simulink library "Contact_Forces_Lib"  (R2018a)
settings: Solver=ode45  StartTime=0.0  StopTime=10.0  RelTol=1e-3  EnableMultiTasking=on
undefined symbols (not defined in the file or in its folder): b_contact, custom_param_1, custom_param_2, k_contact, l_cone, length_cylinder, length_tube, mu_kinetic, mu_static, pen_exponent, pen_full_damp_F, rad_s_cone, radius_cylinder, radius_tube, v_thr, X, Y, Z
libraries: nesl_utility x153, sm_lib x64, $bdroot x53, simulink x9, fl_lib x1
(part 3 of 7)

== system Contact_Forces_Lib/2D/Circle to Circle Force/Fn ==
  note: Resolve Normal Force in
      | Circle F reference frame
  note: Resolve Normal Force in
      | Circle B reference frame
  Fn : Inport
  R : Inport  Port=2
  azm : Inport  Port=3
  Fn in CirB : Subsystem
  Fn in CirF : Subsystem
  FxCirF : Outport
  FyCirF : Outport  Port=2
  FxCirB : Outport  Port=3
  FyCirB : Outport  Port=4
  wires:
  Fn in CirF/2(FxCirF) -> FxCirF/1
  Fn in CirF/1(FyCirF) -> FyCirF/1
  R/1 -> Fn in CirF/1(R)
  azm/1 -> Fn in CirB/2(azm)
  Fn/1 -> Fn in CirB/1(Fn)
  Fn in CirB/2(FyCirB) -> FyCirB/1, Fn in CirF/3(FyCirB)
  Fn in CirB/1(FxCirB) -> Fn in CirF/2(FxCirB), FxCirB/1

== system Contact_Forces_Lib/2D/Circle to Circle Force/Sensing ==
  PS-Simulink Converter1 : nesl_utility/PS-Simulink Converter  PhysicalDomain=network_engine_domain  SubClassName=ps_output  LeftPortType=input  RightPortType=output  PseudoPeriodic=off  Frequencies=[]  Unit=deg  AffineConversion=off
  PS-Simulink Converter{2..7} (6 alike) : nesl_utility/PS-Simulink Converter  PhysicalDomain=network_engine_domain  SubClassName=ps_output  LeftPortType=input  RightPortType=output  PseudoPeriodic=off  Frequencies=[]  Unit=1  AffineConversion=off
  Selector : Selector  NumberOfDimensions=2  InputPortWidth=3  IndexOptions=Index vector (dialog),Index vector (dialog)  Indices=[1,2],[1,2]  OutputSizes=1,1
  Transform Sensor Base : sm_lib/Frames and Transforms/Transform Sensor  MeasurementFrame=Base  SenseAngle=off  SenseAxis=off  SenseAngle1=off  SenseAngle2=off  SenseAngle3=off  SenseQ=off  SenseR=on  SenseOmegaX=off  SenseOmegaY=off  SenseOmegaZ=off  SenseOmega1=off  SenseOmega2=off  SenseOmega3=off  SenseQDot=off  SenseRDot=off  SenseAlphaX=off  SenseAlphaY=off  SenseAlphaZ=off  SenseAlpha1=off  SenseAlpha2=off  SenseAlpha3=off  SenseQDDot=off  SenseRDDot=off  SenseX=off  SenseY=off  SenseZ=off  SenseRad=on  SenseAzim=on  SenseDist=off  SenseInc=off  SenseXDot=off  SenseYDot=off  SenseZDot=off  SenseRadDot=on  SenseAzimDot=off  SenseDistDot=off  SenseIncDot=off  SenseXDDot=off  SenseYDDot=off  SenseZDDot=off  SenseRadDDot=off  SenseAzimDDot=off  SenseDistDDot=off  SenseIncDDot=off  BlockFunction=simmechanics.library.frames_transforms.transform_sensor
  Transform Sensor NonRotBase : sm_lib/Frames and Transforms/Transform Sensor  MeasurementFrame=NonRotatingBase  SenseAngle=off  SenseAxis=off  SenseAngle1=off  SenseAngle2=off  SenseAngle3=off  SenseQ=off  SenseR=off  SenseOmegaX=off  SenseOmegaY=off  SenseOmegaZ=off  SenseOmega1=off  SenseOmega2=off  SenseOmega3=off  SenseQDot=off  SenseRDot=off  SenseAlphaX=off  SenseAlphaY=off  SenseAlphaZ=off  SenseAlpha1=off  SenseAlpha2=off  SenseAlpha3=off  SenseQDDot=off  SenseRDDot=off  SenseX=off  SenseY=off  SenseZ=off  SenseRad=off  SenseAzim=off  SenseDist=off  SenseInc=off  SenseXDot=off  SenseYDot=off  SenseZDot=off  SenseRadDot=off  SenseAzimDot=on  SenseDistDot=off  SenseIncDot=off  SenseXDDot=off  SenseYDDot=off  SenseZDDot=off  SenseRadDDot=off  SenseAzimDDot=off  SenseDistDDot=off  SenseIncDDot=off  BlockFunction=simmechanics.library.frames_transforms.transform_sensor
  Transform Sensor WorldB : sm_lib/Frames and Transforms/Transform Sensor  MeasurementFrame=Follower  SenseAngle=off  SenseAxis=off  SenseAngle1=off  SenseAngle2=off  SenseAngle3=off  SenseQ=off  SenseR=off  SenseOmegaX=off  SenseOmegaY=off  SenseOmegaZ=on  SenseOmega1=off  SenseOmega2=off  SenseOmega3=off  SenseQDot=off  SenseRDot=off  SenseAlphaX=off  SenseAlphaY=off  SenseAlphaZ=off  SenseAlpha1=off  SenseAlpha2=off  SenseAlpha3=off  SenseQDDot=off  SenseRDDot=off  SenseX=off  SenseY=off  SenseZ=off  SenseRad=off  SenseAzim=off  SenseDist=off  SenseInc=off  SenseXDot=off  SenseYDot=off  SenseZDot=off  SenseRadDot=off  SenseAzimDot=off  SenseDistDot=off  SenseIncDot=off  SenseXDDot=off  SenseYDDot=off  SenseZDDot=off  SenseRadDDot=off  SenseAzimDDot=off  SenseDistDDot=off  SenseIncDDot=off  BlockFunction=simmechanics.library.frames_transforms.transform_sensor
  Transform Sensor WorldF : sm_lib/Frames and Transforms/Transform Sensor  MeasurementFrame=Follower  SenseAngle=off  SenseAxis=off  SenseAngle1=off  SenseAngle2=off  SenseAngle3=off  SenseQ=off  SenseR=off  SenseOmegaX=off  SenseOmegaY=off  SenseOmegaZ=on  SenseOmega1=off  SenseOmega2=off  SenseOmega3=off  SenseQDot=off  SenseRDot=off  SenseAlphaX=off  SenseAlphaY=off  SenseAlphaZ=off  SenseAlpha1=off  SenseAlpha2=off  SenseAlpha3=off  SenseQDDot=off  SenseRDDot=off  SenseX=off  SenseY=off  SenseZ=off  SenseRad=off  SenseAzim=off  SenseDist=off  SenseInc=off  SenseXDot=off  SenseYDot=off  SenseZDot=off  SenseRadDot=off  SenseAzimDot=off  SenseDistDot=off  SenseIncDot=off  SenseXDDot=off  SenseYDDot=off  SenseZDDot=off  SenseRadDDot=off  SenseAzimDDot=off  SenseDistDDot=off  SenseIncDDot=off  BlockFunction=simmechanics.library.frames_transforms.transform_sensor
  World Frame1 : sm_lib/Frames and Transforms/World Frame  BlockFunction=simmechanics.library.frames_transforms.world_frame
  F : PMIOPort  Side=Left
  B : PMIOPort  Port=2  Side=Left
  rad : Outport
  vrad : Outport  Port=2
  azm : Outport  Port=3
  vazm : Outport  Port=4
  wzf : Outport  Port=5
  wzb : Outport  Port=6
  R : Outport  Port=7
  wires:
  PS-Simulink Converter7/1 -> wzb/1
  PS-Simulink Converter1/1 -> azm/1
  PS-Simulink Converter5/1 -> rad/1
  PS-Simulink Converter4/1 -> vrad/1
  Selector/1 -> R/1
  PS-Simulink Converter6/1 -> Selector/1
  PS-Simulink Converter2/1 -> vazm/1
  PS-Simulink Converter3/1 -> wzf/1
  connections:
  PS-Simulink Converter7/LConn1 -- Transform Sensor WorldB/RConn2
  Transform Sensor WorldF/LConn1 -- Transform Sensor WorldB/LConn1 -- World Frame1/RConn1
  PS-Simulink Converter4/LConn1 -- Transform Sensor Base/RConn5
  PS-Simulink Converter5/LConn1 -- Transform Sensor Base/RConn3
  PS-Simulink Converter1/LConn1 -- Transform Sensor Base/RConn4
  PS-Simulink Converter6/LConn1 -- Transform Sensor Base/RConn2
  Transform Sensor Base/LConn1 -- B/RConn1 -- Transform Sensor NonRotBase/LConn1 -- Transform Sensor WorldB/RConn1
  Transform Sensor WorldF/RConn1 -- F/RConn1 -- Transform Sensor Base/RConn1 -- Transform Sensor NonRotBase/RConn1
  PS-Simulink Converter2/LConn1 -- Transform Sensor NonRotBase/RConn2
  PS-Simulink Converter3/LConn1 -- Transform Sensor WorldF/RConn2

== system Contact_Forces_Lib/2D/Circle to Circle Force/Sum ==
  FnxCirF : Inport
  FnyCirF : Inport  Port=2
  FnxCirB : Inport  Port=3
  FnyCirB : Inport  Port=4
  FfxCirF : Inport  Port=5
  FfyCirF : Inport  Port=6
  FfxCirB : Inport  Port=7
  FfyCirB : Inport  Port=8
  TzCirF : Inport  Port=9
  TzCirB : Inport  Port=10
  Simulink-PS Converter{,3..7} (6 alike) : nesl_utility/Simulink-PS Converter  PhysicalDomain=network_engine_domain  SubClassName=ps_input  LeftPortType=input  RightPortType=output  PseudoPeriodic=off  Frequencies=[]  NoiseDistribution=none  NoiseParameters=[]  Unit=1  AffineConversion=off  InputFiltering=off  SimscapeFilterOrder=1  InputFilterTimeConstant=.001  UdotUserProvided=[]
  Sum{2..5} (4 alike) : Sum
  FxF : PMIOPort  Side=Right
  FyF : PMIOPort  Port=2  Side=Right
  TzF : PMIOPort  Port=3  Side=Right
  FxB : PMIOPort  Port=4  Side=Right
  FyB : PMIOPort  Port=5  Side=Right
  TzB : PMIOPort  Port=6  Side=Right
  wires:
  FfxCirF/1 -> Sum4/2
  FfyCirF/1 -> Sum2/2
  FfyCirB/1 -> Sum5/2
  FfxCirB/1 -> Sum3/2
  TzCirF/1 -> Simulink-PS Converter6/1
  TzCirB/1 -> Simulink-PS Converter7/1
  FnxCirF/1 -> Sum4/1
  FnyCirF/1 -> Sum2/1
  FnxCirB/1 -> Sum3/1
  FnyCirB/1 -> Sum5/1
  Sum4/1 -> Simulink-PS Converter/1
  Sum2/1 -> Simulink-PS Converter3/1
  Sum3/1 -> Simulink-PS Converter4/1
  Sum5/1 -> Simulink-PS Converter5/1
  connections:
  Simulink-PS Converter/RConn1 -- FxF/RConn1
  Simulink-PS Converter3/RConn1 -- FyF/RConn1
  Simulink-PS Converter4/RConn1 -- FxB/RConn1
  Simulink-PS Converter5/RConn1 -- FyB/RConn1
  Simulink-PS Converter6/RConn1 -- TzF/RConn1
  Simulink-PS Converter7/RConn1 -- TzB/RConn1

== system Contact_Forces_Lib/2D/Circle to Circle Force Enabled/Calculate Penetration ==
  rad : Inport
  vrad : Inport  Port=2
  Constant : Constant  Value=cirF_rad+cirB_rad
  Dead Zone : DeadZone  LowerValue=-inf  UpperValue=0  SaturateOnIntegerOverflow=on
  Gain2 : Gain  Gain=-1
  Sum1 : Sum  Inputs=+-
  Pen : Outport
  Pen Vel : Outport  Port=2
  wires:
  vrad/1 -> Gain2/1
  Gain2/1 -> Pen Vel/1
  Dead Zone/1 -> Pen/1
  Sum1/1 -> Dead Zone/1
  Constant/1 -> Sum1/1
  rad/1 -> Sum1/2

== system Contact_Forces_Lib/2D/Circle to Circle Force Enabled/Ff ==
  Fn : Inport
  azm : Inport  Port=2
  Pen : Inport  Port=3
  rad : Inport  Port=4
  vazm : Inport  Port=5
  wzf : Inport  Port=6
  wzb : Inport  Port=7
  R : Inport  Port=8
  Friction Law : $bdroot/Friction Law  OverrideUsingVariant=None
  Resolve Ff : Subsystem
  vTan : Subsystem
  FxCirF : Outport
  FyCirF : Outport  Port=2
  FxCirB : Outport  Port=3
  FyCirB : Outport  Port=4
  TzCirF : Outport  Port=5
  TzCirB : Outport  Port=6
  Ff : Outport  Port=7
  wires:
  Resolve Ff/6(TzCirB) -> TzCirB/1
  Resolve Ff/5(TzCirF) -> TzCirF/1
  Resolve Ff/2(FyCirB) -> FyCirB/1
  Resolve Ff/1(FxCirB) -> FxCirB/1
  Resolve Ff/3(FyCirF) -> FyCirF/1
  Resolve Ff/4(FxCirF) -> FxCirF/1
  Friction Law/1 -> Ff/1, Resolve Ff/2(Ff)
  vTan/1(vTan) -> Friction Law/2
  wzf/1 -> vTan/4(wzf)
  vazm/1 -> vTan/3(vazm)
  rad/1 -> vTan/1(rad)
  Fn/1 -> Friction Law/1
  Pen/1 -> vTan/2(Pen)
  azm/1 -> Resolve Ff/3(azm)
  R/1 -> Resolve Ff/1(R)
  wzb/1 -> vTan/5(wzb)

== system Contact_Forces_Lib/2D/Circle to Circle Force Enabled/Fn ==
  note: Resolve Normal Force in
      | Circle B reference frame
  note: Resolve Normal Force in
      | Circle F reference frame
  Fn : Inport
  R : Inport  Port=2
  azm : Inport  Port=3
  Fn in CirB : Subsystem
  Fn in CirF : Subsystem
  FxCirF : Outport
  FyCirF : Outport  Port=2
  FxCirB : Outport  Port=3
  FyCirB : Outport  Port=4
  wires:
  Fn in CirB/1(FxCirB) -> FxCirB/1, Fn in CirF/2(FxCirB)
  Fn in CirB/2(FyCirB) -> Fn in CirF/3(FyCirB), FyCirB/1
  Fn/1 -> Fn in CirB/1(Fn)
  azm/1 -> Fn in CirB/2(azm)
  R/1 -> Fn in CirF/1(R)
  Fn in CirF/1(FyCirF) -> FyCirF/1
  Fn in CirF/2(FxCirF) -> FxCirF/1

== system Contact_Forces_Lib/2D/Circle to Circle Force Enabled/Sensing ==
  PS-Simulink Converter1 : nesl_utility/PS-Simulink Converter  PhysicalDomain=network_engine_domain  SubClassName=ps_output  LeftPortType=input  RightPortType=output  PseudoPeriodic=off  Frequencies=[]  Unit=deg  AffineConversion=off
  PS-Simulink Converter{2..7} (6 alike) : nesl_utility/PS-Simulink Converter  PhysicalDomain=network_engine_domain  SubClassName=ps_output  LeftPortType=input  RightPortType=output  PseudoPeriodic=off  Frequencies=[]  Unit=1  AffineConversion=off
  Selector : Selector  NumberOfDimensions=2  InputPortWidth=3  IndexOptions=Index vector (dialog),Index vector (dialog)  Indices=[1,2],[1,2]  OutputSizes=1,1
  Transform Sensor Base : sm_lib/Frames and Transforms/Transform Sensor  MeasurementFrame=Base  SenseAngle=off  SenseAxis=off  SenseAngle1=off  SenseAngle2=off  SenseAngle3=off  SenseQ=off  SenseR=on  SenseOmegaX=off  SenseOmegaY=off  SenseOmegaZ=off  SenseOmega1=off  SenseOmega2=off  SenseOmega3=off  SenseQDot=off  SenseRDot=off  SenseAlphaX=off  SenseAlphaY=off  SenseAlphaZ=off  SenseAlpha1=off  SenseAlpha2=off  SenseAlpha3=off  SenseQDDot=off  SenseRDDot=off  SenseX=off  SenseY=off  SenseZ=off  SenseRad=on  SenseAzim=on  SenseDist=off  SenseInc=off  SenseXDot=off  SenseYDot=off  SenseZDot=off  SenseRadDot=on  SenseAzimDot=off  SenseDistDot=off  SenseIncDot=off  SenseXDDot=off  SenseYDDot=off  SenseZDDot=off  SenseRadDDot=off  SenseAzimDDot=off  SenseDistDDot=off  SenseIncDDot=off  BlockFunction=simmechanics.library.frames_transforms.transform_sensor
  Transform Sensor NonRotBase : sm_lib/Frames and Transforms/Transform Sensor  MeasurementFrame=NonRotatingBase  SenseAngle=off  SenseAxis=off  SenseAngle1=off  SenseAngle2=off  SenseAngle3=off  SenseQ=off  SenseR=off  SenseOmegaX=off  SenseOmegaY=off  SenseOmegaZ=off  SenseOmega1=off  SenseOmega2=off  SenseOmega3=off  SenseQDot=off  SenseRDot=off  SenseAlphaX=off  SenseAlphaY=off  SenseAlphaZ=off  SenseAlpha1=off  SenseAlpha2=off  SenseAlpha3=off  SenseQDDot=off  SenseRDDot=off  SenseX=off  SenseY=off  SenseZ=off  SenseRad=off  SenseAzim=off  SenseDist=off  SenseInc=off  SenseXDot=off  SenseYDot=off  SenseZDot=off  SenseRadDot=off  SenseAzimDot=on  SenseDistDot=off  SenseIncDot=off  SenseXDDot=off  SenseYDDot=off  SenseZDDot=off  SenseRadDDot=off  SenseAzimDDot=off  SenseDistDDot=off  SenseIncDDot=off  BlockFunction=simmechanics.library.frames_transforms.transform_sensor
  Transform Sensor WorldB : sm_lib/Frames and Transforms/Transform Sensor  MeasurementFrame=Follower  SenseAngle=off  SenseAxis=off  SenseAngle1=off  SenseAngle2=off  SenseAngle3=off  SenseQ=off  SenseR=off  SenseOmegaX=off  SenseOmegaY=off  SenseOmegaZ=on  SenseOmega1=off  SenseOmega2=off  SenseOmega3=off  SenseQDot=off  SenseRDot=off  SenseAlphaX=off  SenseAlphaY=off  SenseAlphaZ=off  SenseAlpha1=off  SenseAlpha2=off  SenseAlpha3=off  SenseQDDot=off  SenseRDDot=off  SenseX=off  SenseY=off  SenseZ=off  SenseRad=off  SenseAzim=off  SenseDist=off  SenseInc=off  SenseXDot=off  SenseYDot=off  SenseZDot=off  SenseRadDot=off  SenseAzimDot=off  SenseDistDot=off  SenseIncDot=off  SenseXDDot=off  SenseYDDot=off  SenseZDDot=off  SenseRadDDot=off  SenseAzimDDot=off  SenseDistDDot=off  SenseIncDDot=off  BlockFunction=simmechanics.library.frames_transforms.transform_sensor
  Transform Sensor WorldF : sm_lib/Frames and Transforms/Transform Sensor  MeasurementFrame=Follower  SenseAngle=off  SenseAxis=off  SenseAngle1=off  SenseAngle2=off  SenseAngle3=off  SenseQ=off  SenseR=off  SenseOmegaX=off  SenseOmegaY=off  SenseOmegaZ=on  SenseOmega1=off  SenseOmega2=off  SenseOmega3=off  SenseQDot=off  SenseRDot=off  SenseAlphaX=off  SenseAlphaY=off  SenseAlphaZ=off  SenseAlpha1=off  SenseAlpha2=off  SenseAlpha3=off  SenseQDDot=off  SenseRDDot=off  SenseX=off  SenseY=off  SenseZ=off  SenseRad=off  SenseAzim=off  SenseDist=off  SenseInc=off  SenseXDot=off  SenseYDot=off  SenseZDot=off  SenseRadDot=off  SenseAzimDot=off  SenseDistDot=off  SenseIncDot=off  SenseXDDot=off  SenseYDDot=off  SenseZDDot=off  SenseRadDDot=off  SenseAzimDDot=off  SenseDistDDot=off  SenseIncDDot=off  BlockFunction=simmechanics.library.frames_transforms.transform_sensor
  World Frame1 : sm_lib/Frames and Transforms/World Frame  BlockFunction=simmechanics.library.frames_transforms.world_frame
  F : PMIOPort  Side=Left
  B : PMIOPort  Port=2  Side=Left
  rad : Outport
  vrad : Outport  Port=2
  azm : Outport  Port=3
  vazm : Outport  Port=4
  wzf : Outport  Port=5
  wzb : Outport  Port=6
  R : Outport  Port=7
  wires:
  PS-Simulink Converter3/1 -> wzf/1
  PS-Simulink Converter2/1 -> vazm/1
  PS-Simulink Converter6/1 -> Selector/1
  Selector/1 -> R/1
  PS-Simulink Converter4/1 -> vrad/1
  PS-Simulink Converter5/1 -> rad/1
  PS-Simulink Converter1/1 -> azm/1
  PS-Simulink Converter7/1 -> wzb/1
  connections:
  PS-Simulink Converter3/LConn1 -- Transform Sensor WorldF/RConn2
  PS-Simulink Converter2/LConn1 -- Transform Sensor NonRotBase/RConn2
  Transform Sensor NonRotBase/RConn1 -- Transform Sensor Base/RConn1 -- F/RConn1 -- Transform Sensor WorldF/RConn1
  Transform Sensor WorldB/RConn1 -- Transform Sensor NonRotBase/LConn1 -- B/RConn1 -- Transform Sensor Base/LConn1
  PS-Simulink Converter6/LConn1 -- Transform Sensor Base/RConn2
  PS-Simulink Converter1/LConn1 -- Transform Sensor Base/RConn4
  PS-Simulink Converter5/LConn1 -- Transform Sensor Base/RConn3
  PS-Simulink Converter4/LConn1 -- Transform Sensor Base/RConn5
  World Frame1/RConn1 -- Transform Sensor WorldB/LConn1 -- Transform Sensor WorldF/LConn1
  PS-Simulink Converter7/LConn1 -- Transform Sensor WorldB/RConn2

== system Contact_Forces_Lib/2D/Circle to Circle Force Enabled/Sum ==
  FnxCirF : Inport
  FnyCirF : Inport  Port=2
  FnxCirB : Inport  Port=3
  FnyCirB : Inport  Port=4
  FfxCirF : Inport  Port=5
  FfyCirF : Inport  Port=6
  FfxCirB : Inport  Port=7
  FfyCirB : Inport  Port=8
  TzCirF : Inport  Port=9
  TzCirB : Inport  Port=10
  Simulink-PS Converter{,3..7} (6 alike) : nesl_utility/Simulink-PS Converter  PhysicalDomain=network_engine_domain  SubClassName=ps_input  LeftPortType=input  RightPortType=output  PseudoPeriodic=off  Frequencies=[]  NoiseDistribution=none  NoiseParameters=[]  Unit=1  AffineConversion=off  InputFiltering=off  SimscapeFilterOrder=1  InputFilterTimeConstant=.001  UdotUserProvided=[]
  Sum{2..5} (4 alike) : Sum
  FxF : PMIOPort  Side=Right
  FyF : PMIOPort  Port=2  Side=Right
  TzF : PMIOPort  Port=3  Side=Right
  FxB : PMIOPort  Port=4  Side=Right
  FyB : PMIOPort  Port=5  Side=Right
  TzB : PMIOPort  Port=6  Side=Right
  wires:
  Sum5/1 -> Simulink-PS Converter5/1
  Sum3/1 -> Simulink-PS Converter4/1
  Sum2/1 -> Simulink-PS Converter3/1
  Sum4/1 -> Simulink-PS Converter/1
  FnyCirB/1 -> Sum5/1
  FnxCirB/1 -> Sum3/1
  FnyCirF/1 -> Sum2/1
  FnxCirF/1 -> Sum4/1
  TzCirB/1 -> Simulink-PS Converter7/1
  TzCirF/1 -> Simulink-PS Converter6/1
  FfxCirB/1 -> Sum3/2
  FfyCirB/1 -> Sum5/2
  FfyCirF/1 -> Sum2/2
  FfxCirF/1 -> Sum4/2
  connections:
  Simulink-PS Converter7/RConn1 -- TzB/RConn1
  Simulink-PS Converter6/RConn1 -- TzF/RConn1
  Simulink-PS Converter5/RConn1 -- FyB/RConn1
  Simulink-PS Converter4/RConn1 -- FxB/RConn1
  Simulink-PS Converter3/RConn1 -- FyF/RConn1
  Simulink-PS Converter/RConn1 -- FxF/RConn1

== system Contact_Forces_Lib/2D/Circle to Finite Line Force/Calculate Penetration ==
  x : Inport
  vx : Inport  Port=2
  Abs : Abs  ZeroCross=off
  Constant : Constant  Value=circle_rad+line_depth
  Dead Zone : DeadZone  LowerValue=-inf  UpperValue=0  SaturateOnIntegerOverflow=on
  Gain2 : Gain  Gain=-1
  Product : Product
  Sign vx : Signum  ZeroCross=off
  Sign x : Signum  ZeroCross=off
  Sum : Sum  Inputs=+-
  Pos Sign : Outport
  Pen : Outport  Port=2
  Pen Vel : Outport  Port=3
  Vel Sign : Outport  Port=4
  wires:
  Gain2/1 -> Pen Vel/1
  Dead Zone/1 -> Pen/1
  Product/1 -> Gain2/1
  Sign vx/1 -> Vel Sign/1
  Sign x/1 -> Product/1, Pos Sign/1
  Abs/1 -> Sum/2
  Sum/1 -> Dead Zone/1
  Constant/1 -> Sum/1
  vx/1 -> Sign vx/1, Product/2
  x/1 -> Abs/1, Sign x/1

== system Contact_Forces_Lib/2D/Circle to Finite Line Force/Demux ==
  F : Inport
  Bus Creator : BusCreator  Inputs=2
  Bus Creator1 : BusCreator  Inputs=3
  Constant : Constant  Value=0
  Demux : Demux  Outputs=[3 3]
  Demux1 : Demux  Outputs=3
  Demux2 : Demux  Outputs=3
  Gain : Gain  Gain=-1
  Gain1 : Gain
  Simulink-PS Converter{,1..7} (8 alike) : nesl_utility/Simulink-PS Converter  PhysicalDomain=network_engine_domain  SubClassName=ps_input  LeftPortType=input  RightPortType=output  PseudoPeriodic=off  Frequencies=[]  NoiseDistribution=none  NoiseParameters=[]  Unit=1  AffineConversion=off  InputFiltering=off  SimscapeFilterOrder=1  InputFilterTimeConstant=.001  UdotUserProvided=[]
  Fx Cir : PMIOPort  Side=Right
  Fy Cir : PMIOPort  Port=2  Side=Right
  Fz Cir : PMIOPort  Port=3  Side=Right
  Tz Cir : PMIOPort  Port=4  Side=Right
  Fx Lin : PMIOPort  Port=5  Side=Right
  Fy Lin : PMIOPort  Port=6  Side=Right
  Fz Lin : PMIOPort  Port=7  Side=Right
  Tz Lin : PMIOPort  Port=8  Side=Right
  FCir : Outport
  FLin : Outport  Port=2
  wires:
  Gain/1 -> Demux2/1
  Demux1/3 -> Simulink-PS Converter7/1
  Demux2/3 -> Bus Creator1/3, Simulink-PS Converter6/1  "Tz"
  Demux2/1 -> Bus Creator1/1, Simulink-PS Converter3/1  "Fx"
  Demux2/2 -> Bus Creator1/2, Simulink-PS Converter4/1  "Fy"
  Constant/1 -> Simulink-PS Converter5/1, Simulink-PS Converter2/1
  Demux1/2 -> Bus Creator/2, Simulink-PS Converter1/1  "Fy"
  Demux1/1 -> Bus Creator/1, Simulink-PS Converter/1  "Fx"
  Demux/1 -> Gain1/1
  Demux/2 -> Gain/1
  F/1 -> Demux/1
  Gain1/1 -> Demux1/1
  Bus Creator/1 -> FCir/1  "FCir"
  Bus Creator1/1 -> FLin/1  "FLin"
  connections:
  Tz Cir/RConn1 -- Simulink-PS Converter7/RConn1
  Fz Lin/RConn1 -- Simulink-PS Converter5/RConn1
  Fy Lin/RConn1 -- Simulink-PS Converter4/RConn1
  Fx Lin/RConn1 -- Simulink-PS Converter3/RConn1
  Tz Lin/RConn1 -- Simulink-PS Converter6/RConn1
  Fx Cir/RConn1 -- Simulink-PS Converter/RConn1
  Fy Cir/RConn1 -- Simulink-PS Converter1/RConn1
  Fz Cir/RConn1 -- Simulink-PS Converter2/RConn1

== system Contact_Forces_Lib/2D/Circle to Finite Line Force/Enable Force ==
  y : Inport
  Abs1 : Abs  ZeroCross=off
  Activation limit for contact force : Constant  Value=line_length/2
  Sum : Sum  Inputs=+-
  Enable : Outport
  wires:
  Sum/1 -> Enable/1
  Activation limit for contact force/1 -> Sum/1
  y/1 -> Abs1/1
  Abs1/1 -> Sum/2

== system Contact_Forces_Lib/2D/Circle to Finite Line Force/Forces ==
  M arm : Inport
  X Sep : Inport  Port=2
  Pos Cmp : Inport  Port=3
  Pen : Inport  Port=4
  Vel : Inport  Port=5
  Vel_Cmp : Inport  Port=6
  Unit Vector : Inport  Port=7
  vy : Inport  Port=8
  wz : Inport  Port=9
  Action Port : ActionPort
  Force Law : $bdroot/Force Law  OverrideUsingVariant=Linear
  Mux : Mux  Inputs=6
  Resolve Forces : Subsystem
  Subsystem : Subsystem
  Fnf : Outport  InitialOutput=[0]
  F : Outport  Port=2
  wires:
  X Sep/1 -> Resolve Forces/3(X Sep)
  Force Law/2 -> Resolve Forces/5(Damp Force Mag)
  Force Law/1 -> Resolve Forces/4(Spr Force Mag)
  Resolve Forces/3(Tz Cir) -> Mux/3
  vy/1 -> Resolve Forces/8(vy)
  wz/1 -> Resolve Forces/9(wz)
  Unit Vector/1 -> Resolve Forces/7(Unit Vector)
  Vel_Cmp/1 -> Resolve Forces/6(Vel Cmp)
  Mux/1 -> F/1
  Pos Cmp/1 -> Resolve Forces/2(Pos Cmp)
  M arm/1 -> Resolve Forces/1(Moment arm)
  Resolve Forces/2(Fy Cir) -> Mux/2
  Resolve Forces/1(Fx Cir) -> Mux/1
  Resolve Forces/6(Tz Lin) -> Mux/6
  Resolve Forces/5(Fy Lin) -> Mux/5
  Vel/1 -> Force Law/2
  Pen/1 -> Force Law/1
  Resolve Forces/4(Fx Lin) -> Mux/4
  Resolve Forces/7(Fn) -> Subsystem/1(Fn)
  Resolve Forces/8(Ff) -> Subsystem/2(Ff)
  Subsystem/1(Out) -> Fnf/1

== system Contact_Forces_Lib/2D/Circle to Finite Line Force/No Force ==
  Action Port : ActionPort
  Zeros : Constant  Value=[0 0 0 0 0 0]  SampleTime=0
  Zeros1 : Constant  Value=[0 0]  SampleTime=0
  Fnf : Outport  InitialOutput=[0]
  F : Outport  Port=2  InitialOutput=[0 0 0 0 0 0]
  wires:
  Zeros/1 -> F/1
  Zeros1/1 -> Fnf/1

== system Contact_Forces_Lib/2D/Circle to Finite Line Force/Sensing ==
  PS-Simulink Converter{,1..4,6} (6 alike) : nesl_utility/PS-Simulink Converter  PhysicalDomain=network_engine_domain  SubClassName=ps_output  LeftPortType=input  RightPortType=output  PseudoPeriodic=off  Frequencies=[]  Unit=1  AffineConversion=off
  Scope : Scope
  Scope1 : Scope  NumInputPorts=2
  Selector : Selector  NumberOfDimensions=2  InputPortWidth=3  IndexOptions=Index vector (dialog),Index vector (dialog)  Indices=[1],[1,2]  OutputSizes=1,1
  Transform Sensor : sm_lib/Frames and Transforms/Transform Sensor  MeasurementFrame=Base  SenseAngle=off  SenseAxis=off  SenseAngle1=off  SenseAngle2=off  SenseAngle3=off  SenseQ=off  SenseR=off  SenseOmegaX=off  SenseOmegaY=off  SenseOmegaZ=on  SenseOmega1=off  SenseOmega2=off  SenseOmega3=off  SenseQDot=off  SenseRDot=off  SenseAlphaX=off  SenseAlphaY=off  SenseAlphaZ=off  SenseAlpha1=off  SenseAlpha2=off  SenseAlpha3=off  SenseQDDot=off  SenseRDDot=off  SenseX=on  SenseY=on  SenseZ=off  SenseRad=off  SenseAzim=off  SenseDist=off  SenseInc=off  SenseXDot=on  SenseYDot=on  SenseZDot=off  SenseRadDot=off  SenseAzimDot=off  SenseDistDot=off  SenseIncDot=off  SenseXDDot=off  SenseYDDot=off  SenseZDDot=off  SenseRadDDot=off  SenseAzimDDot=off  SenseDistDDot=off  SenseIncDDot=off  BlockFunction=simmechanics.library.frames_transforms.transform_sensor
  Transform Sensor1 : sm_lib/Frames and Transforms/Transform Sensor  MeasurementFrame=World  SenseAngle=off  SenseAxis=off  SenseAngle1=off  SenseAngle2=off  SenseAngle3=off  SenseQ=off  SenseR=on  SenseOmegaX=off  SenseOmegaY=off  SenseOmegaZ=off  SenseOmega1=off  SenseOmega2=off  SenseOmega3=off  SenseQDot=off  SenseRDot=off  SenseAlphaX=off  SenseAlphaY=off  SenseAlphaZ=off  SenseAlpha1=off  SenseAlpha2=off  SenseAlpha3=off  SenseQDDot=off  SenseRDDot=off  SenseX=off  SenseY=off  SenseZ=off  SenseRad=off  SenseAzim=off  SenseDist=off  SenseInc=off  SenseXDot=off  SenseYDot=off  SenseZDot=off  SenseRadDot=off  SenseAzimDot=off  SenseDistDot=off  SenseIncDot=off  SenseXDDot=off  SenseYDDot=off  SenseZDDot=off  SenseRadDDot=off  SenseAzimDDot=off  SenseDistDDot=off  SenseIncDDot=off  BlockFunction=simmechanics.library.frames_transforms.transform_sensor
  F : PMIOPort  Side=Left
  B : PMIOPort  Port=2  Side=Left
  y : Outport
  x : Outport  Port=2
  vx : Outport  Port=3
  q : Outport  Port=4
  vy : Outport  Port=5
  wz : Outport  Port=6
  wires:
  PS-Simulink Converter4/1 -> wz/1
  Selector/1 -> q/1, Scope/1
  PS-Simulink Converter6/1 -> Selector/1
  PS-Simulink Converter3/1 -> vy/1
  PS-Simulink Converter2/1 -> vx/1
  PS-Simulink Converter1/1 -> y/1, Scope1/2
  PS-Simulink Converter/1 -> x/1, Scope1/1
  connections:
  PS-Simulink Converter3/LConn1 -- Transform Sensor/RConn6
  PS-Simulink Converter6/LConn1 -- Transform Sensor1/RConn2
  PS-Simulink Converter2/LConn1 -- Transform Sensor/RConn5
  PS-Simulink Converter1/LConn1 -- Transform Sensor/RConn4
  PS-Simulink Converter/LConn1 -- Transform Sensor/RConn3
  PS-Simulink Converter4/LConn1 -- Transform Sensor/RConn2
  Transform Sensor1/LConn1 -- B/RConn1 -- Transform Sensor/LConn1
  Transform Sensor1/RConn1 -- F/RConn1 -- Transform Sensor/RConn1

== system Contact_Forces_Lib/2D/Circle to Finite Line Force Enabled/Calculate Penetration ==
  x : Inport
  vx : Inport  Port=2
  Abs : Abs  ZeroCross=off
  Constant : Constant  Value=circle_rad+line_depth
  Dead Zone : DeadZone  LowerValue=-inf  UpperValue=0  SaturateOnIntegerOverflow=on
  Gain2 : Gain  Gain=-1
  Product : Product
  Sign vx : Signum  ZeroCross=off
  Sign x : Signum  ZeroCross=off
  Sum : Sum  Inputs=+-
  Pos Sign : Outport
  Pen : Outport  Port=2
  Pen Vel : Outport  Port=3
  Vel Sign : Outport  Port=4
  wires:
  x/1 -> Sign x/1, Abs/1
  vx/1 -> Product/2, Sign vx/1
  Constant/1 -> Sum/1
  Sum/1 -> Dead Zone/1
  Abs/1 -> Sum/2
  Sign x/1 -> Pos Sign/1, Product/1
  Sign vx/1 -> Vel Sign/1
  Product/1 -> Gain2/1
  Dead Zone/1 -> Pen/1
  Gain2/1 -> Pen Vel/1

== system Contact_Forces_Lib/2D/Circle to Finite Line Force Enabled/Demux ==
  F : Inport
  Bus Creator : BusCreator  Inputs=2
  Bus Creator1 : BusCreator  Inputs=3
  Constant : Constant  Value=0
  Demux : Demux  Outputs=[3 3]
  Demux1 : Demux  Outputs=3
  Demux2 : Demux  Outputs=3
  Gain : Gain  Gain=-1
  Gain1 : Gain
  Simulink-PS Converter{,1..7} (8 alike) : nesl_utility/Simulink-PS Converter  PhysicalDomain=network_engine_domain  SubClassName=ps_input  LeftPortType=input  RightPortType=output  PseudoPeriodic=off  Frequencies=[]  NoiseDistribution=none  NoiseParameters=[]  Unit=1  AffineConversion=off  InputFiltering=off  SimscapeFilterOrder=1  InputFilterTimeConstant=.001  UdotUserProvided=[]
  Fx Cir : PMIOPort  Side=Right
  Fy Cir : PMIOPort  Port=2  Side=Right
  Fz Cir : PMIOPort  Port=3  Side=Right
  Tz Cir : PMIOPort  Port=4  Side=Right
  Fx Lin : PMIOPort  Port=5  Side=Right
  Fy Lin : PMIOPort  Port=6  Side=Right
  Fz Lin : PMIOPort  Port=7  Side=Right
  Tz Lin : PMIOPort  Port=8  Side=Right
  FCir : Outport
  FLin : Outport  Port=2
  wires:
  Bus Creator1/1 -> FLin/1  "FLin"
  Bus Creator/1 -> FCir/1  "FCir"
  Gain1/1 -> Demux1/1
  F/1 -> Demux/1
  Demux/2 -> Gain/1
  Demux/1 -> Gain1/1
  Demux1/1 -> Simulink-PS Converter/1, Bus Creator/1  "Fx"
  Demux1/2 -> Simulink-PS Converter1/1, Bus Creator/2  "Fy"
  Constant/1 -> Simulink-PS Converter2/1, Simulink-PS Converter5/1
  Demux2/2 -> Simulink-PS Converter4/1, Bus Creator1/2  "Fy"
  Demux2/1 -> Simulink-PS Converter3/1, Bus Creator1/1  "Fx"
  Demux2/3 -> Simulink-PS Converter6/1, Bus Creator1/3  "Tz"
  Demux1/3 -> Simulink-PS Converter7/1
  Gain/1 -> Demux2/1
  connections:
  Fz Cir/RConn1 -- Simulink-PS Converter2/RConn1
  Fy Cir/RConn1 -- Simulink-PS Converter1/RConn1
  Fx Cir/RConn1 -- Simulink-PS Converter/RConn1
  Tz Lin/RConn1 -- Simulink-PS Converter6/RConn1
  Fx Lin/RConn1 -- Simulink-PS Converter3/RConn1
  Fy Lin/RConn1 -- Simulink-PS Converter4/RConn1
  Fz Lin/RConn1 -- Simulink-PS Converter5/RConn1
  Tz Cir/RConn1 -- Simulink-PS Converter7/RConn1

== system Contact_Forces_Lib/2D/Circle to Finite Line Force Enabled/Enable Force ==
  y : Inport
  Abs1 : Abs  ZeroCross=off
  Activation limit for contact force : Constant  Value=line_length/2
  Sum : Sum  Inputs=+-
  Enable : Outport
  wires:
  Abs1/1 -> Sum/2
  y/1 -> Abs1/1
  Activation limit for contact force/1 -> Sum/1
  Sum/1 -> Enable/1

== system Contact_Forces_Lib/2D/Circle to Finite Line Force Enabled/Forces ==
  M arm : Inport
  X Sep : Inport  Port=2
  Pos Cmp : Inport  Port=3
  Pen : Inport  Port=4
  Vel : Inport  Port=5
  Vel_Cmp : Inport  Port=6
  Unit Vector : Inport  Port=7
  vy : Inport  Port=8
  wz : Inport  Port=9
  Action Port : ActionPort  ActionType=then
  Force Law : $bdroot/Force Law  OverrideUsingVariant=Linear
  Mux : Mux  Inputs=6
  Resolve Forces : Subsystem
  Subsystem : Subsystem
  Fnf : Outport  InitialOutput=[0]
  F : Outport  Port=2
  wires:
  Subsystem/1(Out) -> Fnf/1
  Resolve Forces/8(Ff) -> Subsystem/2(Ff)
  Resolve Forces/7(Fn) -> Subsystem/1(Fn)
  Resolve Forces/4(Fx Lin) -> Mux/4
  Pen/1 -> Force Law/1
  Vel/1 -> Force Law/2
  Resolve Forces/5(Fy Lin) -> Mux/5
  Resolve Forces/6(Tz Lin) -> Mux/6
  Resolve Forces/1(Fx Cir) -> Mux/1
  Resolve Forces/2(Fy Cir) -> Mux/2
  M arm/1 -> Resolve Forces/1(Moment arm)
  Pos Cmp/1 -> Resolve Forces/2(Pos Cmp)
  Mux/1 -> F/1
  Vel_Cmp/1 -> Resolve Forces/6(Vel Cmp)
  Unit Vector/1 -> Resolve Forces/7(Unit Vector)
  wz/1 -> Resolve Forces/9(wz)
  vy/1 -> Resolve Forces/8(vy)
  Resolve Forces/3(Tz Cir) -> Mux/3
  Force Law/1 -> Resolve Forces/4(Spr Force Mag)
  Force Law/2 -> Resolve Forces/5(Damp Force Mag)
  X Sep/1 -> Resolve Forces/3(X Sep)

== system Contact_Forces_Lib/2D/Circle to Finite Line Force Enabled/No Force ==
  Action Port : ActionPort  ActionType=else
  Zeros : Constant  Value=[0 0 0 0 0 0]  SampleTime=0
  Zeros1 : Constant  Value=[0 0]  SampleTime=0
  Fnf : Outport  InitialOutput=[0]
  F : Outport  Port=2  InitialOutput=[0 0 0 0 0 0]
  wires:
  Zeros1/1 -> Fnf/1
  Zeros/1 -> F/1

== system Contact_Forces_Lib/2D/Circle to Finite Line Force Enabled/Sensing ==
  In : Inport
  Bus Selector : BusSelector  OutputSignals=vy
  PS-Simulink Converter{,1..4,6} (6 alike) : nesl_utility/PS-Simulink Converter  PhysicalDomain=network_engine_domain  SubClassName=ps_output  LeftPortType=input  RightPortType=output  PseudoPeriodic=off  Frequencies=[]  Unit=1  AffineConversion=off
  Product : Product
  Selector : Selector  NumberOfDimensions=2  InputPortWidth=3  IndexOptions=Index vector (dialog),Index vector (dialog)  Indices=[1],[1,2]  OutputSizes=1,1
  Sign : Signum  ZeroCross=off
  Sum : Sum  Inputs=|+-
  Transform Sensor : sm_lib/Frames and Transforms/Transform Sensor  MeasurementFrame=Base  SenseAngle=off  SenseAxis=off  SenseAngle1=off  SenseAngle2=off  SenseAngle3=off  SenseQ=off  SenseR=off  SenseOmegaX=off  SenseOmegaY=off  SenseOmegaZ=on  SenseOmega1=off  SenseOmega2=off  SenseOmega3=off  SenseQDot=off  SenseRDot=off  SenseAlphaX=off  SenseAlphaY=off  SenseAlphaZ=off  SenseAlpha1=off  SenseAlpha2=off  SenseAlpha3=off  SenseQDDot=off  SenseRDDot=off  SenseX=on  SenseY=on  SenseZ=off  SenseRad=off  SenseAzim=off  SenseDist=off  SenseInc=off  SenseXDot=on  SenseYDot=on  SenseZDot=off  SenseRadDot=off  SenseAzimDot=off  SenseDistDot=off  SenseIncDot=off  SenseXDDot=off  SenseYDDot=off  SenseZDDot=off  SenseRadDDot=off  SenseAzimDDot=off  SenseDistDDot=off  SenseIncDDot=off  BlockFunction=simmechanics.library.frames_transforms.transform_sensor
  Transform Sensor1 : sm_lib/Frames and Transforms/Transform Sensor  MeasurementFrame=World  SenseAngle=off  SenseAxis=off  SenseAngle1=off  SenseAngle2=off  SenseAngle3=off  SenseQ=off  SenseR=on  SenseOmegaX=off  SenseOmegaY=off  SenseOmegaZ=off  SenseOmega1=off  SenseOmega2=off  SenseOmega3=off  SenseQDot=off  SenseRDot=off  SenseAlphaX=off  SenseAlphaY=off  SenseAlphaZ=off  SenseAlpha1=off  SenseAlpha2=off  SenseAlpha3=off  SenseQDDot=off  SenseRDDot=off  SenseX=off  SenseY=off  SenseZ=off  SenseRad=off  SenseAzim=off  SenseDist=off  SenseInc=off  SenseXDot=off  SenseYDot=off  SenseZDot=off  SenseRadDot=off  SenseAzimDot=off  SenseDistDot=off  SenseIncDot=off  SenseXDDot=off  SenseYDDot=off  SenseZDDot=off  SenseRadDDot=off  SenseAzimDDot=off  SenseDistDDot=off  SenseIncDDot=off  BlockFunction=simmechanics.library.frames_transforms.transform_sensor
  F : PMIOPort  Side=Left
  B : PMIOPort  Port=2  Side=Left
  y : Outport
  x : Outport  Port=2
  vx : Outport  Port=3
  q : Outport  Port=4
  vy : Outport  Port=5
  wz : Outport  Port=6
  wires:
  PS-Simulink Converter/1 -> Sign/1, x/1
  PS-Simulink Converter1/1 -> y/1
  PS-Simulink Converter2/1 -> vx/1
  PS-Simulink Converter3/1 -> Sum/1
  PS-Simulink Converter6/1 -> Selector/1
  Selector/1 -> q/1
  PS-Simulink Converter4/1 -> wz/1
  Sum/1 -> vy/1
  In/1 -> Bus Selector/1
  Bus Selector/1 -> Product/2  "<vy>"
  Sign/1 -> Product/1
  Product/1 -> Sum/2
  connections:
  Transform Sensor/RConn1 -- F/RConn1 -- Transform Sensor1/RConn1
  Transform Sensor/LConn1 -- B/RConn1 -- Transform Sensor1/LConn1
  PS-Simulink Converter4/LConn1 -- Transform Sensor/RConn2
  PS-Simulink Converter/LConn1 -- Transform Sensor/RConn3
  PS-Simulink Converter1/LConn1 -- Transform Sensor/RConn4
  PS-Simulink Converter2/LConn1 -- Transform Sensor/RConn5
  PS-Simulink Converter6/LConn1 -- Transform Sensor1/RConn2
  PS-Simulink Converter3/LConn1 -- Transform Sensor/RConn6

== system Contact_Forces_Lib/2D/Circle to Hole Force/Calculate Penetration ==
  Pos : Inport
  Vel : Inport  Port=2
  Constant : Constant  Value=max_frame_sep
  Dead Zone Outside : DeadZone  LowerValue=-inf  UpperValue=0  SaturateOnIntegerOverflow=on
  Gain2 : Gain  Gain=-1
  Sum1 : Sum  Inputs=|-+
  Pen : Outport
  Pen Vel : Outport  Port=2
  wires:
  Pos/1 -> Sum1/1
  Sum1/1 -> Dead Zone Outside/1
  Constant/1 -> Sum1/2
  Dead Zone Outside/1 -> Pen/1
  Gain2/1 -> Pen Vel/1
  Vel/1 -> Gain2/1

== system Contact_Forces_Lib/2D/Circle to Hole Force/Sensing ==
  PS-Simulink Converter1 : nesl_utility/PS-Simulink Converter  PhysicalDomain=network_engine_domain  SubClassName=ps_output  LeftPortType=input  RightPortType=output  PseudoPeriodic=off  Frequencies=[]  Unit=deg  AffineConversion=off
  PS-Simulink Converter4 : nesl_utility/PS-Simulink Converter  PhysicalDomain=network_engine_domain  SubClassName=ps_output  LeftPortType=input  RightPortType=output  PseudoPeriodic=off  Frequencies=[]  Unit=1  AffineConversion=off
  PS-Simulink Converter5 : nesl_utility/PS-Simulink Converter  PhysicalDomain=network_engine_domain  SubClassName=ps_output  LeftPortType=input  RightPortType=output  PseudoPeriodic=off  Frequencies=[]  Unit=1  AffineConversion=off
  PS-Simulink Converter6 : nesl_utility/PS-Simulink Converter  PhysicalDomain=network_engine_domain  SubClassName=ps_output  LeftPortType=input  RightPortType=output  PseudoPeriodic=off  Frequencies=[]  Unit=1  AffineConversion=off
  Selector : Selector  NumberOfDimensions=2  InputPortWidth=3  IndexOptions=Index vector (dialog),Index vector (dialog)  Indices=[1],[1,2]  OutputSizes=1,1
  Transform Sensor : sm_lib/Frames and Transforms/Transform Sensor  MeasurementFrame=NonRotatingBase  SenseAngle=off  SenseAxis=off  SenseAngle1=off  SenseAngle2=off  SenseAngle3=off  SenseQ=off  SenseR=off  SenseOmegaX=off  SenseOmegaY=off  SenseOmegaZ=off  SenseOmega1=off  SenseOmega2=off  SenseOmega3=off  SenseQDot=off  SenseRDot=off  SenseAlphaX=off  SenseAlphaY=off  SenseAlphaZ=off  SenseAlpha1=off  SenseAlpha2=off  SenseAlpha3=off  SenseQDDot=off  SenseRDDot=off  SenseX=off  SenseY=off  SenseZ=off  SenseRad=on  SenseAzim=on  SenseDist=off  SenseInc=off  SenseXDot=off  SenseYDot=off  SenseZDot=off  SenseRadDot=on  SenseAzimDot=off  SenseDistDot=off  SenseIncDot=off  SenseXDDot=off  SenseYDDot=off  SenseZDDot=off  SenseRadDDot=off  SenseAzimDDot=off  SenseDistDDot=off  SenseIncDDot=off  BlockFunction=simmechanics.library.frames_transforms.transform_sensor
  Transform Sensor1 : sm_lib/Frames and Transforms/Transform Sensor  MeasurementFrame=World  SenseAngle=off  SenseAxis=off  SenseAngle1=off  SenseAngle2=off  SenseAngle3=off  SenseQ=off  SenseR=on  SenseOmegaX=off  SenseOmegaY=off  SenseOmegaZ=off  SenseOmega1=off  SenseOmega2=off  SenseOmega3=off  SenseQDot=off  SenseRDot=off  SenseAlphaX=off  SenseAlphaY=off  SenseAlphaZ=off  SenseAlpha1=off  SenseAlpha2=off  SenseAlpha3=off  SenseQDDot=off  SenseRDDot=off  SenseX=off  SenseY=off  SenseZ=off  SenseRad=off  SenseAzim=off  SenseDist=off  SenseInc=off  SenseXDot=off  SenseYDot=off  SenseZDot=off  SenseRadDot=off  SenseAzimDot=off  SenseDistDot=off  SenseIncDot=off  SenseXDDot=off  SenseYDDot=off  SenseZDDot=off  SenseRadDDot=off  SenseAzimDDot=off  SenseDistDDot=off  SenseIncDDot=off  BlockFunction=simmechanics.library.frames_transforms.transform_sensor
  F : PMIOPort  Side=Left
  B : PMIOPort  Port=2  Side=Left
  rad : Outport
  vrad : Outport  Port=2
  q : Outport  Port=3
  azm : Outport  Port=4
  wires:
  PS-Simulink Converter1/1 -> azm/1
  PS-Simulink Converter5/1 -> rad/1
  PS-Simulink Converter4/1 -> vrad/1
  Selector/1 -> q/1
  PS-Simulink Converter6/1 -> Selector/1
  connections:
  PS-Simulink Converter4/LConn1 -- Transform Sensor/RConn4
  PS-Simulink Converter5/LConn1 -- Transform Sensor/RConn2
  PS-Simulink Converter1/LConn1 -- Transform Sensor/RConn3
  PS-Simulink Converter6/LConn1 -- Transform Sensor1/RConn2
  Transform Sensor1/LConn1 -- B/RConn1 -- Transform Sensor/LConn1
  Transform Sensor1/RConn1 -- Transform Sensor/RConn1 -- F/RConn1

== system Contact_Forces_Lib/2D/Circle to Ring Force/Check Active Range ==
  azm : Inport
  " Upper Bound" : simulink/Logic and Bit Operations/Compare To Constant  relop=<=  const=active_angle(2)  OutDataTypeStr=boolean  ZeroCross=off
  Logical Operator : Logic  AllPortsSameDT=off  OutDataTypeStr=boolean
  Lower Bound : simulink/Logic and Bit Operations/Compare To Constant  relop=>=  const=active_angle(1)  OutDataTypeStr=boolean  ZeroCross=off
  En : Outport
  wires:
  azm/1 -> " Upper Bound"/1, Lower Bound/1
  " Upper Bound"/1 -> Logical Operator/1
  Logical Operator/1 -> En/1
  Lower Bound/1 -> Logical Operator/2

== system Contact_Forces_Lib/2D/Circle to Ring Force/Forces ==
  rad : Inport
  vrad : Inport  Port=2
  azm : Inport  Port=3
  vazm : Inport  Port=4
  wzf : Inport  Port=5
  R : Inport  Port=6
  Action Port : ActionPort
  Bus Creator : BusCreator  Inputs=6
  Calculate Penetration : Subsystem
  Ff : Subsystem
  Fn : Subsystem
  Force Law : $bdroot/Force Law  OverrideUsingVariant=Linear
  Gain1 : Gain  Gain=-1
  Mux : Mux  Inputs=6
  Product : Product
  Sum : Subsystem
  Sum1 : Sum  Inputs=+-
  Frc : Outport
  Out : Outport  Port=2  InitialOutput=[0]
  wires:
  Bus Creator/1 -> Out/1
  Force Law/1 -> Bus Creator/4, Sum1/1  "Spr Force"
  Calculate Penetration/3(Pen Vel) -> Bus Creator/1, Force Law/2  "Penetration Vel"
  vrad/1 -> Calculate Penetration/2(vrad)
  rad/1 -> Ff/7(rad), Calculate Penetration/1(rad)
  Product/1 -> Bus Creator/5, Gain1/1  "Normal Force"
  Calculate Penetration/2(Pen) -> Bus Creator/2, Ff/6(Pen), Force Law/1  "Penetration"
  Calculate Penetration/1(sign) -> Product/1
  Force Law/2 -> Bus Creator/3, Sum1/2  "Damp Force"
  Sum1/1 -> Product/2
  Gain1/1 -> Ff/5(Fn), Fn/1(Fn)
  R/1 -> Ff/1(R), Fn/2(R)
  azm/1 -> Fn/3(azm), Ff/2(azm)
  vazm/1 -> Ff/3(vazm)
  wzf/1 -> Ff/4(wzf)
  Fn/1(FxCirF) -> Sum/1(FnxCirF)
  Fn/2(FyCirF) -> Sum/2(FnyCirF)
  Fn/3(FxCirB) -> Sum/3(FnxCirB)
  Fn/4(FyCirB) -> Sum/4(FnyCirB)
  Ff/4(FyCirB) -> Sum/8(FfyCirB)
  Ff/6(TzCirB) -> Sum/10(TzCirB)
  Ff/3(FxCirB) -> Sum/7(FfxCirB)
  Ff/5(TzCirF) -> Sum/9(TzCirF)
  Ff/1(FxCirF) -> Sum/5(FfxCirF)
  Ff/2(FyCirF) -> Sum/6(FfyCirF)
  Sum/2(FyF) -> Mux/2
  Sum/3(TzF) -> Mux/3
  Sum/1(FxF) -> Mux/1
  Sum/5(FyB) -> Mux/5
  Sum/4(FxB) -> Mux/4
  Sum/6(TzB) -> Mux/6
  Mux/1 -> Frc/1
  Ff/7(Ff) -> Bus Creator/6  "Friction Force"

== system Contact_Forces_Lib/2D/Circle to Ring Force/No Force ==
  Action Port : ActionPort
  Zeros : Constant  Value=[0 0 0 0 0 0]  SampleTime=0
  F : Outport  InitialOutput=[0]
  wires:
  Zeros/1 -> F/1

== system Contact_Forces_Lib/2D/Circle to Ring Force/Sensing ==
  PS-Simulink Converter1 : nesl_utility/PS-Simulink Converter  PhysicalDomain=network_engine_domain  SubClassName=ps_output  LeftPortType=input  RightPortType=output  PseudoPeriodic=off  Frequencies=[]  Unit=deg  AffineConversion=off
  PS-Simulink Converter{2..6} (5 alike) : nesl_utility/PS-Simulink Converter  PhysicalDomain=network_engine_domain  SubClassName=ps_output  LeftPortType=input  RightPortType=output  PseudoPeriodic=off  Frequencies=[]  Unit=1  AffineConversion=off
  Selector : Selector  NumberOfDimensions=2  InputPortWidth=3  IndexOptions=Index vector (dialog),Index vector (dialog)  Indices=[1,2],[1,2]  OutputSizes=1,1
  Transform Sensor Base : sm_lib/Frames and Transforms/Transform Sensor  MeasurementFrame=Base  SenseAngle=off  SenseAxis=off  SenseAngle1=off  SenseAngle2=off  SenseAngle3=off  SenseQ=off  SenseR=on  SenseOmegaX=off  SenseOmegaY=off  SenseOmegaZ=off  SenseOmega1=off  SenseOmega2=off  SenseOmega3=off  SenseQDot=off  SenseRDot=off  SenseAlphaX=off  SenseAlphaY=off  SenseAlphaZ=off  SenseAlpha1=off  SenseAlpha2=off  SenseAlpha3=off  SenseQDDot=off  SenseRDDot=off  SenseX=off  SenseY=off  SenseZ=off  SenseRad=on  SenseAzim=on  SenseDist=off  SenseInc=off  SenseXDot=off  SenseYDot=off  SenseZDot=off  SenseRadDot=on  SenseAzimDot=on  SenseDistDot=off  SenseIncDot=off  SenseXDDot=off  SenseYDDot=off  SenseZDDot=off  SenseRadDDot=off  SenseAzimDDot=off  SenseDistDDot=off  SenseIncDDot=off  BlockFunction=simmechanics.library.frames_transforms.transform_sensor
  Transform Sensor World : sm_lib/Frames and Transforms/Transform Sensor  MeasurementFrame=Follower  SenseAngle=off  SenseAxis=off  SenseAngle1=off  SenseAngle2=off  SenseAngle3=off  SenseQ=off  SenseR=off  SenseOmegaX=off  SenseOmegaY=off  SenseOmegaZ=on  SenseOmega1=off  SenseOmega2=off  SenseOmega3=off  SenseQDot=off  SenseRDot=off  SenseAlphaX=off  SenseAlphaY=off  SenseAlphaZ=off  SenseAlpha1=off  SenseAlpha2=off  SenseAlpha3=off  SenseQDDot=off  SenseRDDot=off  SenseX=off  SenseY=off  SenseZ=off  SenseRad=off  SenseAzim=off  SenseDist=off  SenseInc=off  SenseXDot=off  SenseYDot=off  SenseZDot=off  SenseRadDot=off  SenseAzimDot=off  SenseDistDot=off  SenseIncDot=off  SenseXDDot=off  SenseYDDot=off  SenseZDDot=off  SenseRadDDot=off  SenseAzimDDot=off  SenseDistDDot=off  SenseIncDDot=off  BlockFunction=simmechanics.library.frames_transforms.transform_sensor
  World Frame : sm_lib/Frames and Transforms/World Frame  BlockFunction=simmechanics.library.frames_transforms.world_frame
  F : PMIOPort  Side=Left
  B : PMIOPort  Port=2  Side=Left
  rad : Outport
  vrad : Outport  Port=2
  azm : Outport  Port=3
  vazm : Outport  Port=4
  wzf : Outport  Port=5
  R : Outport  Port=6
  wires:
  PS-Simulink Converter3/1 -> wzf/1
  PS-Simulink Converter2/1 -> vazm/1
  PS-Simulink Converter6/1 -> Selector/1
  Selector/1 -> R/1
  PS-Simulink Converter4/1 -> vrad/1
  PS-Simulink Converter5/1 -> rad/1
  PS-Simulink Converter1/1 -> azm/1
  connections:
  World Frame/RConn1 -- Transform Sensor World/LConn1
  PS-Simulink Converter3/LConn1 -- Transform Sensor World/RConn2
  PS-Simulink Converter2/LConn1 -- Transform Sensor Base/RConn6
  Transform Sensor Base/RConn1 -- Transform Sensor World/RConn1 -- F/RConn1
  Transform Sensor Base/LConn1 -- B/RConn1
  PS-Simulink Converter6/LConn1 -- Transform Sensor Base/RConn2
  PS-Simulink Converter1/LConn1 -- Transform Sensor Base/RConn4
  PS-Simulink Converter5/LConn1 -- Transform Sensor Base/RConn3
  PS-Simulink Converter4/LConn1 -- Transform Sensor Base/RConn5

== system Contact_Forces_Lib/2D/Circle to Ring Force/Subsystem ==
  Frc : Inport
  Demux : Demux  Outputs=6
  Simulink-PS Converter{,1..5} (6 alike) : nesl_utility/Simulink-PS Converter  PhysicalDomain=network_engine_domain  SubClassName=ps_input  LeftPortType=input  RightPortType=output  PseudoPeriodic=off  Frequencies=[]  NoiseDistribution=none  NoiseParameters=[]  Unit=1  AffineConversion=off  InputFiltering=off  SimscapeFilterOrder=1  InputFilterTimeConstant=0.001  UdotUserProvided=1
  FxF : PMIOPort  Side=Right
  FyF : PMIOPort  Port=2  Side=Right
  TzF : PMIOPort  Port=3  Side=Right
  FxB : PMIOPort  Port=4  Side=Right
  FyB : PMIOPort  Port=5  Side=Right
  TzB : PMIOPort  Port=6  Side=Right
  wires:
  Frc/1 -> Demux/1
  Demux/6 -> Simulink-PS Converter5/1
  Demux/5 -> Simulink-PS Converter4/1
  Demux/4 -> Simulink-PS Converter3/1
  Demux/3 -> Simulink-PS Converter2/1
  Demux/1 -> Simulink-PS Converter/1
  Demux/2 -> Simulink-PS Converter1/1
  connections:
  Simulink-PS Converter2/RConn1 -- TzF/RConn1
  Simulink-PS Converter4/RConn1 -- FyB/RConn1
  Simulink-PS Converter3/RConn1 -- FxB/RConn1
  Simulink-PS Converter5/RConn1 -- TzB/RConn1
  Simulink-PS Converter/RConn1 -- FxF/RConn1
  Simulink-PS Converter1/RConn1 -- FyF/RConn1

== system Contact_Forces_Lib/2D/Composite Forces/Box to Belt Force ==
  Spd : Inport
  Add2 : Sum
  Belt Ends : Subsystem
      mask Display:
      | image(imread('Box_to_Belt_Ends_IMAGE.jpg'));
      | port_label('LConn',1,'Bel');
      | port_label('RConn',1,'Box');
      | port_label('input',1,'In');
      | port_label('output',1,'Fn');
  Belt Faces : Subsystem
      mask Display:
      | image(imread('Box_to_Belt_Faces_IMAGE.jpg'));
      | port_label('LConn',1,'Bel');
      | port_label('RConn',1,'Box');
      | port_label('input',1,'In');
      | port_label('output',1,'Fn');
  Bus Creator : BusCreator  Inputs=2
  Enable : Constant
  Box : PMIOPort  Side=Right
  Bel : PMIOPort  Port=2  Side=Left
  Fn : Outport
  wires:
  Belt Faces/1(Fn) -> Add2/1
  Belt Ends/1(Fn) -> Add2/2
  Add2/1 -> Fn/1
  Enable/1 -> Bus Creator/1  "Enable"
  Spd/1 -> Bus Creator/2  "vy"
  Bus Creator/1 -> Belt Ends/1(In), Belt Faces/1(In1)
  connections:
  Belt Faces/LConn1 -- Bel/RConn1 -- Belt Ends/LConn1
  Belt Faces/RConn1 -- Box/RConn1 -- Belt Ends/RConn1

== system Contact_Forces_Lib/2D/Composite Forces/Box to Box Force ==
  Abs : Abs  ZeroCross=off
  Abs1 : Abs  ZeroCross=off
  Add : Sum
  BoxB Corners : Subsystem  mask(Contact Forces, Base Box Corners){}
      mask help:
      | This subsystem models planar contact forces the corners of the Follower box and the faces of the Base Box.
      |
      | Click the Help button for a diagram of the contact forces and the parameters.
      mask Help: web(which('Box_to_Box_Contact_Forces_BoxB_Corners.html'));
      mask Display:
      | image(imread('BoxB_Corners_IMAGE.jpg'));
      | port_label('LConn',1,'BoxB');
      | port_label('RConn',1,'BoxF');
  BoxF Corners : Subsystem  mask(Contact Forces, Follower Box Corners){}
      mask help:
      | This subsystem models planar contact forces the corners of the Follower box and the faces of the Base Box.
      |
      | Click the Help button for a diagram of the contact forces and the parameters.
      mask Help: web(which('Box_to_Box_Contact_Forces_BoxF_Corners.html'));
      mask Display:
      | image(imread('BoxF_Corners_IMAGE.jpg'));
      | port_label('LConn',1,'BoxB');
      | port_label('RConn',1,'BoxF');
  Goto Tag Visibility : GotoTagVisibility  GotoTag=FrcFC
  Goto Tag Visibility1 : GotoTagVisibility  GotoTag=FrcBC
  Sum of Elements : Sum  Inputs=+
  Sum of Elements1 : Sum  Inputs=+
  BoxF : PMIOPort  Side=Left
  BoxB : PMIOPort  Port=2  Side=Right
  tag scope: Forces=global
  wires:
  Sum of Elements1/1 -> Add/2
  Add/1 -> [Forces]
  Abs1/1 -> Sum of Elements1/1
  [FrcBC] -> Abs1/1
  Abs/1 -> Sum of Elements/1
  Sum of Elements/1 -> Add/1
  [FrcFC] -> Abs/1
  connections:
  BoxB Corners/LConn1 -- BoxF Corners/LConn1 -- BoxB/RConn1
  BoxB Corners/RConn1 -- BoxF Corners/RConn1 -- BoxF/RConn1
